simulink model "mydct"  (R2018b)
settings: Solver=VariableStepAuto  StartTime=0.0  StopTime=1  RelTol=1e-3
libraries: dspsnks4 x1, dspvision x1
settings Model: Creator=DSP-36  LastModifiedBy=DSP-36

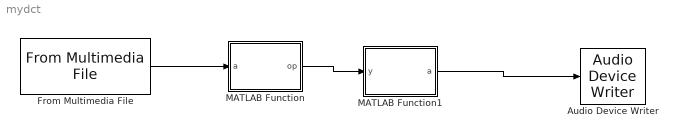
== system mydct ==
  Audio Device Writer : dspsnks4/Audio Device Writer  Driver=DirectSound  Device=Default  InheritSampleRate=on  SampleRate=44100  BitDepth=16-bit integer  BufferSize=4096  NumBuffers=10  DefaultOutputChannelMapping=on  OutputChannelMapping=1:2  OutputNumUnderrunSamples=off  DriverIdx=1  DeviceWarnFlag=''
  From Multimedia File : dspvision/From Multimedia File  inputFilename=C:\Users\DSP-36\Desktop\17ucc038\input.wav  loop=on  numPlays=inf  outputStreams=Audio only  videoDataType=single  audioDataType=double  inheritSampleTime=on  userDefinedSampleTime=1/30  noAudioOutput=off  isIntensityVideo=off  fourcc=RGB  colorVideoFormat=Separate color signals  outputEOF=off  dataOrg=Column-major  audioFrameSize=32000  computeAudioFrameSize=off  outSamplingMode=Sample based
      settings: SourceProductBaseCode=VP
  MATLAB Function : MATLAB Function  TreatAsAtomicUnit=on
  MATLAB Function1 : MATLAB Function  TreatAsAtomicUnit=on
  wires:
  MATLAB Function1/1(a) -> Audio Device Writer/1
  MATLAB Function/1(op) -> MATLAB Function1/1(y)
  From Multimedia File/1 -> MATLAB Function/1(a)

== matlab function mydct/MATLAB Function1 ==
  data: y input; a output
function a = fcn(y)
N = length(y);
x = zeros(N,1);
w =zeros(N,1);
a = zeros(N,1);
for n = 1:N
    x(n) = 0;
    for k = 1:N
        if k==1
            w(k) = 1/sqrt(N);
        else
            w(k) = sqrt(2/N);
        end
        x(n) = x(n) + w(k)*y(k)*cos(pi*((2*n)-1)*(k-1)/(2*N));
    end
end


a = x;

== matlab function mydct/MATLAB Function ==
  data: a input; op output
function op = fcn(a)
N = length(a);
y = zeros(N,1);
w =zeros(N,1);
for k = 1:N
    if k==1
        w(k)=1/sqrt(N);
    else
        w(k)=sqrt(2/N);
    end
    temp=0;
    for n=1:N
        temp=temp+a(n)*cos(pi*((2*n)-1)*(k-1)/(2*N));
    end
    y(k)=w(k)*temp;
end
op = y;
